simulink model "ASM_Traffic_V2X_Complete_Model_2"  (R2019a)
settings: Solver=ode1  StartTime=SIM.tstart.v  StopTime=Inf  FixedStep=SIM.StepSize.v  RelTol=1e-3
PostLoadFcn:
  | if any(exist('dsrtsu_mdlpostloadfcn', 'file') ~= 0), dsrtsu_mdlpostloadfcn('Execute', bdroot); end
  | try, asm_mdl_postloadfcn(bdroot, 'UpdateModel', 2200); catch, disp(lasterr); end,
undefined symbols (not defined in the file): _SensorPnts_1, _SensorPnts_13, _SensorPnts_17, _SensorPnts_21, _SensorPnts_25, _SensorPnts_29, _SensorPnts_33, _SensorPnts_37, _SensorPnts_41, _SensorPnts_45, _SensorPnts_49, _SensorPnts_5, _SensorPnts_53, _SensorPnts_57, _SensorPnts_9, _to_, CPT, G5A, ITS, MDL, rad, s_to_rpm, SIM
libraries: simulink x169, ASM_VehicleDynamics_lib x126, ASM_Traffic_lib x83, ASM_Utils_lib x49, mdbs x45, ASM_Environment_lib x17, dspindex x12, dsaV2xLibraryAux x10, dsmpblib x6, dsaV2xAsn1Library x4, dsaV2xLibrary x4, ASM_BrakeHydraulics_lib x4
(part 1 of 36)
PreSaveFcn:
  | , if any(exist('dsmpb_private', 'file') ~= 0), dsmpb_private('dsmpb_mdlclblib', 'PreSave', bdroot); end,
CloseFcn:
  | , if any(exist('dsmpb_private', 'file') ~= 0), dsmpb_private('dsmpb_mdlclblib', 'Close', bdroot); end,
settings Model: RTICANMMDATA=struct('GeneralSetupData',struct('modelroot','C:\Users\FHAachenHIL\Desktop\7_DS_Config\5_NoAD_New\1_mdldesk\Simulation\Models','generalsettings',struct('filesettings',struct('destfolder',struct('Name','RTICANMM_FILES','Check',1),'buildfolder',struct('Name','.','Check',1),'AbsDestfolder',struct('Name','C:\Users\FHAachenHIL\Desktop\7_DS_Config\5_NoAD_New\1_mdldesk\Simulation\Models\RTICANMM_FILES'),'AbsBuildfolder',struct('Name','C:\Users\FHAachenHIL\Desktop\7_DS_Config\5_NoAD_New\1_mdldesk\Simulation\Models'))),'options',struct('addpaths',1,'rmpaths',1,'addtrcexclusion',logical(1),'cannavigator',struct('checkmonitoring',0),'show_usrtrc',0,'use_usrtrc',0),'advanced',struct('options',ones(1,100)),'MPSetup',{{}},'RTI',struct('Type','DSRT','Ver','4.1','Date','02-May-2019'),'modelname','ASM_Traffic','block','ASM_Traffic'))  RTILINMMDATA=struct('GeneralSetupData',[])  DSRTSU_INTERNAL_MDBS_VER=10  DSRTSU_INTERNAL_FLEXRAYCONFIG=1  DSRTSU_INTERNAL_RTIFLEXRAYCONFIG=110  DSRTSU_INTERNAL_RTIFPGA=130  DSMPB_DATASERVER_ModelPortLibVersion1=8  DSMPB_DATASERVER_DataServerVersion1=6  DSMPB_DATASERVER_DataServerStreamVersion1=3  DSMPB_ID_DATA={'330216',struct('BlockId','b1f7d386-c077-4b6f-815e-9957a38efec6','SignalIds',{{'5954efed-ef67-4b42-89e3-5084b45090a5','46c6c21c-6ef7-4bce-a685-35314e3aeb42'}}),'330217',struct('BlockId','ed5b6760-6c8b-4597-8985-96cc864119f9','SignalIds',{{'627e4e4b-6795-451d-b132-3b35f692e399','cadb769f-493c-4926-8cfc-80c1d7e415e4'}}),'330693',struct('BlockId','84e11fc7-b113-489b-a36d-07b56c01051e','SignalIds',{{'d6ecdace-abd9-47b0-9636-db978f49e505','b381082d-6ce8-44f4-ad20-a88c694d043c','f1171069-3abf-4521-8686-68da12ae8162','f12997fb-13dd-47fb-a199-884124e88373','33a83d4b-34dd-4bb2-a080-c0d96c0e7444','ed9617ed-63e6-4252-841f-8cd256f9a792','c4d94f54-a4e4-4e6b-a3f5-bdd9f29a9d42','15fc0dc5-818d-41b9-9325-316e0087897d','5fc40cf9-a339-4045-adf5-9eb5a647bd91','2c42badf-67b8-4972-b237-b7d847a79e24','2d6ab885-034a-426b-a4d8-331cba00cc0a','83513bad-946f-4b2a-b06e-a5b54ac67582','7f7e93e0-f84b-4ac0-9920-c275b8003985','b171feba-60b8-420b-b0d7-260006587811','f516aac7-9c5c-4744-8cba-64c96d215c0d','9a91ebe5-1c5e-4056-b557-0e0db1076263','7c50508e-1c47-48c8-9676-4fb8df70f5b9','c6d12e17-68fd-48eb-9242-ce387edb3efa','ff46a663-5f34-440b-b3bc-6b93d7652bc7','70c5629e-94fa-4dad-b003-5f0ee91b30d9','864ca5d3-ee15-40fd-9f67-5bde9bd55b65','8c924b41-9569-4218-92a0-ce33cbab6020'}}),'330694',struct('BlockId','a862b2ce-fdfe-464c-a6f1-ee7d5bbd7d76','SignalIds',{{'f2281447-8dd6-4b87-a3fd-ba757601a6a3','ed6577a0-1bef-4f93-882d-9a91ba3803b9','f5072a04-e2e8-432a-9d22-5e39f1b004c4','f9be402e-ef68-469d-9a5b-51e341e63153','1a6fa1c0-c78d-4bef-9fa9-3949581777f9','434f5ee9-f735-4340-9052-50d203bce394','e2750fce-2507-4a3e-a71c-871616da759c','a78121f1-2d1e-4fc1-9bd3-1e700b95df97','cfd43ada-4b18-4913-87c2-7150350b7745','748ab899-55d6-4599-8033-eefc4cf8692b','9396844c-ddf9-495e-bf4a-e4337b26c01b','5061b213-d7ab-4036-a402-68c9d851f2f7','f74f67c2-0a64-4121-bbfc-28e28bf8e47c','af8173ae-b56e-4181-af22-ab3597f99b45','ab6ffc97-b1da-485b-b261-68785b2ecf74','c89e4028-be19-4be4-8ae4-07a9cfb3f304','45dfa9da-2b41-4994-bfb5-431cbec6d91f','0f4a48ac-0d04-4973-a79b-6dba9191f613','4897f706-738b-48a8-bfa9-4dce5adfb66f','b0c4fe5a-1a55-469a-bfc9-3e5a391b1d28','cee4ed91-4e62-4f16-9db1-8814ccf7c0ec','e77965e1-b7f4-415c-8908-9a91dfd04724','79bd3ed0-ae18-424e-8479-e097ea261fa6','7949adab-96d5-4dfd-97c4-d5cf440e986d','f2ab8de1-88d0-4341-92a1-f4defd2f3f90','bd765ffd-b1df-4d20-b40b-b08ba0baa9bb','147a83a7-172e-4604-bf04-5a0b9f9a69a1','0e989faa-5d6f-437a-9608-bc5915cdfdf7','9a39d9cd-2ac6-4fea-a823-ea5bd99f580f','d9bd35d1-ce0d-4e25-a189-106bd4b9f84a','959e6de5-da96-4cd1-851d-d0057e4456fd','815f072c-0a7f-4fd6-8c30-6c40f700a896','9aee9d69-733b-49cd-a80a-36da2771f58f','c6f90d32-086e-4841-a108-56354959159b','22eea55d-9a77-4830-86d9-89efdace94fd','c76acaa7-4d73-4d33-9929-8168234ee063','008c6442-9318-4b95-b3d4-07b53b0292c2','b9a30481-22be-4824-9a7c-3a367da5f7e5','5e0cc0b3-4c73-42d3-a56f-471d727ce12d','359885a3-4826-4c3f-aa50-e301bb0f4184','d9b051c3-0428-436f-b8e9-eace4c2c4579','64f5c317-cb27-4a4c-a325-cf6357cb844b','7aed38b5-9bc9-415a-b216-13916177e212','02cf0d23-4107-47fd-84c3-b252337a1963','9c33dc05-2142-432c-9611-36045ad6ec16','ecac5224-2058-46c9-8367-a0d51085fe1f','765bb1a7-d023-41a8-903d-a406451af4fc','4f5bc921-bb9b-4516-a2d8-0d46d6edfa0a','0e14b839-d491-4a1e-aee6-f3f5c7d7bb50','18457238-79de-4e3a-b0d5-409821aa4bed','96051f25-1d22-4dec-ba6f-cc499131fb3a','e18ed66a-7425-4928-a383-5204f5397d27','8d75ab57-f5b7-4d53-8d2e-f8c76d8569c5','36687092-25b3-42f9-a75c-3416bb5260bf','4d5e1a10-c54b-4820-9d88-b0136d7cd812','e599ed13-c6b6-48bb-9374-2671a82569d4','e3af4b03-3db2-441e-a0d6-4f276b79ce4b','825e78c5-827a-4970-b8fe-44ed3d477788','2f348dc1-d43d-4671-b1d1-f46cbe87daf1','343e3104-2314-4619-bae1-dd4c090fa7f4','df4bf909-7eb9-4362-a9c5-d81bea227330','98a03783-5fbc-4b9c-9f1c-81a74cb7af6a','78b869f6-02a3-46b3-8c42-971033ba9de4','88004e9a-d91f-47b9-be0c-5672408ac348','189c9c44-5221-417e-8836-60725b723848','af946d2b-57a6-4c2c-b71f-140b6b02e3f2','90df5bec-5be3-41f9-af4b-0493e5795b67','fee887a9-08b2-4953-96dd-4babc6fd5546','380eb70b-fa16-4dfe-9ee9-78d9cb411dc3','8fe8fb63-2564-43be-828c-a9fe295685f8','33c79d6b-d586-49a0-b7f4-4da2ad91c284','ef27260e-aa76-4ab9-ad3c-03633dde9629','16e6a066-1ed3-4b81-aeb3-56afa55c5cd5','b5c7f2f0-3061-4b24-8ee7-62b27506b806','a2f3d904-f536-4b77-b5ff-26007e182bbc','36680f63-c3b8-4f7c-80dd-29cde9b0854b','4673084a-8171-4f71-bcf9-20c0cf4be7ec','9fa3876b-04bc-431e-ad1d-b72f3b83e37a','37709b06-26d1-4f27-8a6e-c8f1f3493499','0a27576c-b094-4959-ae10-24487d3618bf','b94ac14c-7ff3-4bf2-adc1-e7dcf8ef846d','aa040f24-dfe5-430e-9730-a81b7dc3f6ac','90fd4bbc-ec0f-49bd-9db7-b68249f724e1'}}),'331181',struct('BlockId','25fb538d-07fb-4743-a50e-e603533b0f87','SignalIds',{{'5c53568f-464d-4855-ac76-5002436bdbd6','27e61e6d-fb1c-4471-9743-a52ae1b3f7c4'}}),'331182',struct('BlockId','708c40ea-cccc-4db9-ac35-2feb2ef4f622','SignalIds',{{'d81b8d06-2b1c-443c-8694-f188bd9bd534','cf1714a3-1e9a-4a8e-855e-03d4d95ed40a'}})}  ExtModeArmWhenConnect=off  Creator=dSPACE GmbH  LastModifiedBy=FHAachenHIL
settings DataIOCC: SaveFormat=Structure  SignalLoggingSaveFormat=ModelDataLogs  SaveOutput=off  SaveTime=off  ReturnWorkspaceOutputs=off  SignalLoggingName=sigsOut
settings OptimizationCC: BlockReduction=off  BooleanDataType=off  ConditionallyExecuteInputs=off  OptimizeBlockIOStorage=off  BufferReuse=off  GlobalBufferReuse=off  ExpressionFolding=off  ExpressionDepthLimit=2147483647  LocalBlockOutputs=off  InitFltsAndDblsToZero=on  OptimizeDataStoreBuffers=off  BusAssignmentInplaceUpdate=off
settings DebuggingCC: SignalInfNanChecking=warning  SaveWithParameterizedLinksMsg=none  SignalResolutionControl=TryResolveAllWithWarning  InheritedTsInSrcMsg=none  MultiTaskDSMMsg=warning  MultiTaskCondExecSysMsg=none  MultiTaskRateTransMsg=warning  TasksWithSamePriorityMsg=none  CheckMatrixSingularityMsg=warning  FcnCallInpInsideContextMsg=warning  AllowSymbolicDim=off  StateNameClashWarn=warning  StrictBusMsg=ErrorOnBusTreatedAsVector  NonBusSignalsTreatedAsBus=error  SFUnexpectedBacktrackingDiag=warning  SFNoUnconditionalDefaultTransitionDiag=warning  SFExecutionAtInitializationDiag=none  ArithmeticOperatorsInVariantConditions=warning
settings HardwareCC: ProdBitPerPointer=32  ProdBitPerSizeT=32  ProdBitPerPtrDiffT=32  ProdLargestAtomicInteger=Integer  ProdWordSize=32  ProdHWDeviceType=Custom Processor->Custom  TargetIntDivRoundTo=Zero  TargetEndianess=LittleEndian  TargetHWDeviceType=Custom Processor->Custom
settings ModelReferenceCC: PropagateSignalLabelsOutOfModel=off
settings SFSimCC: SimUseLocalCustomCode=off  MATLABDynamicMemAlloc=off
settings RTWCC: SystemTargetFile=dsrt.tlc  GenCodeOnly=on  MakeCommand=make_dsrt  TemplateMakefile=dsrt_default_tmf  Description=dSPACE Run-Time Target (for VEOS and ConfigurationDesk)  RTWVerbose=off  RetainRTWFile=on  RTWUseLocalCustomCode=off
settings CodeAppCC: StateflowObjectComments=on
settings STFCustomTargetCC: ParMdlRefBuildCompliant=on  GRTInterface=off  SystemTargetFile=dsrt.tlc
settings GRTTargetCC: TargetLangStandard=C89/C90 (ANSI)  CompOptLevelCompliant=off  ConcurrentExecutionCompliant=off  CombineOutputUpdateFcns=off  MatFileLogging=off  CPPClassGenCompliant=off  UseToolchainInfoCompliant=off
settings ConfigComp: CovMetricSettings=dw  CovHtmlReporting=on  CovSaveCumulativeToWorkspaceVar=on  CovSaveSingleToWorkspaceVar=on  CovExternalEMLEnable=off  CovSFcnEnable=off

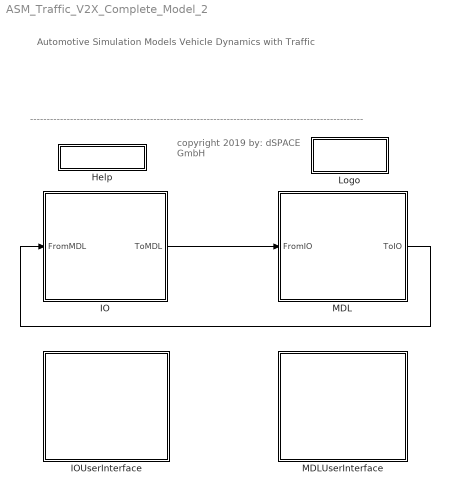
== system ASM_Traffic_V2X_Complete_Model_2 ==
  note: ----------------------------------------------------------------------------------------------------
  note: copyright 2019 by:
      | dSPACE GmbH
  note: Automotive Simulation Models
      | Vehicle Dynamics with Traffic
  Help : Subsystem
      settings: OpenFcn=eval(get_param(gcb,'MaskHelp'))
      mask Help: eval('asm_modelhelp(0,''manual'',''ASMVehicleDynamicsModelDescription.chm'',0)');
      mask Display: fprintf('Help')
  IO : Subsystem
      mask Display: disp('dSPACE\nPeripheral I/O')
  IOUserInterface : Subsystem
      mask Display: disp('User Interface \nfor IO')
  Logo : Subsystem  mask(dSPACE){EmptyParameter=[]}
      mask prompts: EmptyParameter "Mask Parameter 1:"
      settings: OpenFcn=;
      mask Display: image(imread('asm_mdl_dslogo.tif'));
  MDL : Subsystem
      mask Display: disp('Engine + Vehicle\nSimulation Model')
  MDLUserInterface : Subsystem
      mask Display: disp('User Interface \nfor Model')
  wires:
  MDL/1(ToIO) -> IO/1(FromMDL)
  IO/1(ToMDL) -> MDL/1(FromIO)

== system ASM_Traffic_V2X_Complete_Model_2/Help ==
  note: This library can be used for incylinder diesel engine modeling.

== system ASM_Traffic_V2X_Complete_Model_2/IO ==
  FromMDL : Inport
  I/O_Subsystem : Subsystem
      mask Display: image('can2.jpg');
  V2X_Subsystem : Subsystem
      mask Display: image('v2x.jpg');
  ToMDL : Outport
  wires:
  FromMDL/1 -> I/O_Subsystem/1(In1), V2X_Subsystem/1(In1)
  I/O_Subsystem/1(Out1) -> ToMDL/1

== system ASM_Traffic_V2X_Complete_Model_2/IOUserInterface ==
  IO_DISP : Subsystem
      mask Display: disp('Simulation results:\nArbitrary input to\nControlDesk from I/O')
  IO_PAR : Subsystem
      mask Display: disp('Simulation parameters:\nContinuous output from\nControlDesk to I/O')

== system ASM_Traffic_V2X_Complete_Model_2/Logo ==
  note: $Revision: 1.234 $
  note: $Date: 2014/11/26 16:23:07MEZ $
  note: $Workfile: ASM_VehicleDynamics.mdl $

== system ASM_Traffic_V2X_Complete_Model_2/MDL ==
  FromIO : Inport
  Drivetrain : Subsystem
  Engine : Subsystem
  Environment : Subsystem
  MDL_In : Subsystem
  MDL_Out : Subsystem
  SoftECU : Subsystem
  VehicleDynamics : Subsystem
  ToIO : Outport
  wires:
  SoftECU/1(SoftECU_Signals) -> MDL_In/1(from_SoftECU)
  MDL_Out/1(to_IO) -> Environment/1(Vehicle_Signals), SoftECU/1(Vehicle_Signals), ToIO/1
  FromIO/1 -> Environment/2(Input), MDL_In/2(from_IO)
  VehicleDynamics/1(omega_Wheel[FL,FR,RL,RR][rad|s]) -> Drivetrain/3(omega_Wheel[FL,FR,RL,RR][rad|s])
  Drivetrain/2(Trq_Shaft[FL,FR,RL,RR][Nm]) -> VehicleDynamics/1(Trq_Shaft[FL,FR,RL,RR][Nm])
  Engine/1(Trq_Engine[Nm]) -> Drivetrain/1(Trq_Engine[Nm])
  Drivetrain/1(n_Engine[rpm]) -> Engine/2(n_Engine[rpm])
  Environment/1(Environment_Signals) -> VehicleDynamics/2(Environment_Signals), Engine/1(Environment_Signals), SoftECU/2(Environment_Signals), Drivetrain/2(Environment_Signals)

== system ASM_Traffic_V2X_Complete_Model_2/MDLUserInterface ==
  note: --------------------------------- Display Signals and Change Parameters ----------------------------------------------------------------------------------------------------------------------
  note: ----------------------------------------------- MotionDesk 3D-Animation ------------------------------------------------------------
  note: For MotionDesk support replace this block  with the MotionDesk
      | interface from the "ASM_MotionDeskInterface.mdl" which
      | can be found in the "Models" directory.
  note: -------------------- Scope Handling ----------------------
  note: --- Tire Handling ---
  note: --------- Developer/Operator Handling ----------
  note: ----------------------- Project & Experiment Handling -------------------------
  note: ------- Code Generation -------
  note: --- ModelDesk Parameter Group ---
  note: ------- Multi-Instance -------
  ActivateDeveloperVersion : ASM_Utils_lib/Operator/ActivateDeveloperVersion  plotblock_updt=0
  ActivateOperatorVersion : ASM_Utils_lib/Operator/ActivateOperatorVersion  plotblock_updt=0
  Drivetrain : Subsystem
      mask Display: disp('Drivetrain');
  Engine : Subsystem
      mask Display: disp('Engine');
  Environment : Subsystem
      mask Display: disp('Environment');
  GenerateVEOS : ASM_Utils_lib/CodeGeneration/GenerateVEOS
  ModelDeskParaGroupOverview : ASM_Utils_lib/ModelDeskInterface/ModelDeskParaGroupOverview
  ModelDesk_Plotting : Subsystem  Tag=ModelDeskPlottingInterface
      mask Display: disp('ModelDesk Plotting');
  MotionDeskInterface : Subsystem  Tag=MotionDeskInterface
      mask Display: disp('MotionDesk Interface\nSet Configuration Parameters Inside')
  MultiInstanceOverview : ASM_Utils_lib/ModelDeskInterface/MultiInstanceOverview
  OpenExperiment1 : ASM_Utils_lib/OpenExperiment/OpenExperiment  ExpDir=..\Animation\MotionDesk_Traffic\ASMTraffic\ASMTraffic.mdd  dSProduct=MotionDesk
  OpenExperiment2 : ASM_Utils_lib/OpenExperiment/OpenExperiment  ExpDir=..\Parameterization\MOD_Traffic\Experiment_001\Experiment_001.CDE  dSProduct=ModelDesk
  OpenMotionDeskInterfaceModel : Subsystem
      settings: OpenFcn=|
      | InterfaceModel = 'ASM_MotionDeskInterface';
      | 
      | try
      |     open_system(InterfaceModel);                         catch
      |     errordlg(['ERROR opening MotionDesk interface: ',InterfaceModel,'.mdl.']);
      | end
      mask Display: disp('Open\nASM_MotionDeskInterface\nModel')
  ReplaceTireTMEasy : ASM_Utils_lib/BlockReplacement/ReplaceTireTMEasy
  ScopeHandlingGui : ASM_Utils_lib/ReplaceScopes/ScopeHandlingGui
  SoftECU : Subsystem
      mask Display: disp('Soft ECU');
  Toggle_ModelDesk_Plotting : MDLD_Utils_lib/ModelDeskPlotInterface/Toggle_ModelDesk_Plotting  SystemSampleTime=-1
  VehicleDynamics : Subsystem
      mask Display: disp('Vehicle Dynamics');

== system ASM_Traffic_V2X_Complete_Model_2/IO/I//O_Subsystem ==
  note: EGO CAR DATA for CONTROL PC CAN BUS
  note: CAN BUS DATA from CONTROL PC to EGO CAR
  In1 : Inport
  Bus Configuration (1) - In : Subsystem
  Bus Configuration (1) - Out : Subsystem
  Bus Configuration (1)_In : dsmpblib/Data Inport  Priority=10000
      settings: SourceProductName=dSPACE Model Interface Blockset
  Bus Configuration (1)_Out : dsmpblib/Data Outport  Priority=-10000
      settings: SourceProductName=dSPACE Model Interface Blockset
  EgoCar_Command : Subsystem
  EgoCar_Data : Subsystem
  Out1 : Outport
  wires:
  In1/1 -> EgoCar_Data/1(In1), EgoCar_Command/2(In2)
  Bus Configuration (1)_In/1 -> Bus Configuration (1) - Out/1(Out), EgoCar_Command/1(In1)
  EgoCar_Command/1(Out1) -> Out1/1
  Bus Configuration (1) - In/1(In) -> Bus Configuration (1)_Out/1
  EgoCar_Data/1(Out1) -> Bus Configuration (1) - In/1(Input)

== system ASM_Traffic_V2X_Complete_Model_2/IO/V2X_Subsystem ==
  In1 : Inport
  CAM-DENM_Message_Generation : Subsystem
  Car_Data : Subsystem
  Subsystem : Subsystem
  wires:
  Car_Data/1(Output) -> CAM-DENM_Message_Generation/1(Input)
  In1/1 -> Subsystem/1(In1), Car_Data/1(Fellow_Pos_info)

== system ASM_Traffic_V2X_Complete_Model_2/IOUserInterface/IO_DISP ==

== system ASM_Traffic_V2X_Complete_Model_2/IOUserInterface/IO_PAR ==

== system ASM_Traffic_V2X_Complete_Model_2/MDL/Drivetrain ==
  Trq_Engine[Nm] : Inport
  Environment_Signals : Inport  Port=2
  omega_Wheel[FL,FR,RL,RR][rad|s] : Inport  Port=3
  ASMSignalCollector : Subsystem
  Bus Selector1 : BusSelector  OutputSignals=Maneuver.Testbench.n_Engine_Set[rpm],Maneuver.Testbench.SW_Testbench[0Off|1On],Driver.Pos_ClutchPedal[%],Driver.Gear[],Maneuver.MdlControl.Reset_VehicleStates[0|1]
  Bus Selector2 : BusSelector  OutputSignals=Sw_AC[0|1],Ctrl_Lockup_Clutch[%],Gear[]
  Bus Selector3 : BusSelector  OutputSignals=Sw_Starter[0Off|1On]
  Crankshaft : Subsystem  Tag=ASM_CRANKSHAFT
      settings: CopyFcn=asm_blk_copy_gui('start','usecase','crankshaftcopy','drivetrain_variant','flexible')
  DisableReset : Subsystem
      mask Display: disp('DisableReset')
  External Loads : Subsystem
  Final_Drive_Assembly : Subsystem  Tag=ASM_FINAL_DRIVE_ASSEMBLY
      settings: CopyFcn=asm_blk_copy_gui('start','usecase','finaldrivecopy','drivetrain_variant','flexible')
  ModelDesk_MC_ID_Drivetrain : ASM_Utils_lib/ModelDeskInterface/ModelDesk_MC_ID_Drivetrain  Tag=ASM_MAINCOMPONENT  ASMProperties=struct('Name','Drivetrain')
  OpenCrankshaftDemos : Subsystem
      settings: OpenFcn=asm_open_lib('ASM_VehicleDynamics_lib/Drivetrain/Demos_Crankshaft');
      mask Display: disp('Open Demos\nCrankshaft')
  OpenFinalDriveAssemblyDemos : Subsystem
      settings: OpenFcn=asm_open_lib('ASM_VehicleDynamics_lib/Drivetrain/Demos_Final_Drive_Assembly');
      mask Display: disp('Open Demos\nFinal Drive Assembly')
  OpenTransmissionSystemDemos : Subsystem
      settings: OpenFcn=asm_open_lib('ASM_VehicleDynamics_lib/Drivetrain/Demos_Transmission_System');
      mask Display: disp('Open Demos\nTransmission System')
  STARTER : ASM_VehicleDynamics_lib/Drivetrain/Crankshaft_and_Starter/STARTER  Tag=ASM_SUBCOMPONENT  Const_Trq_n0=MDL.Drivetrain.Starter.Const_Trq_n0  Const_n_Trq0=MDL.Drivetrain.Starter.Const_n_Trq0  Const_Inertia_Starter=MDL.Drivetrain.Starter.Const_Inertia_Starter  ASMProperties=struct('Name','STARTER','Version','4.0','Library','ASM_VehicleDynamics_lib')  ASMInstanceName=starter  ASMInstanceID=1
  TEST_BENCH : ASM_VehicleDynamics_lib/Drivetrain/Crankshaft_and_Starter/TEST_BENCH  Tag=ASM_SUBCOMPONENT  Const_P_Gain=MDL.Drivetrain.TestBench.Const_P_Gain  Const_I_Gain=MDL.Drivetrain.TestBench.Const_I_Gain  Const_Trq_Max_TestBench=MDL.Drivetrain.TestBench.Const_Trq_Max_TestBench  Const_Inertia_TestBench=MDL.Drivetrain.TestBench.Const_Inertia_TestBench  StepSize=SIM.StepSize  ASMProperties=struct('Name','TEST_BENCH','Version','2.0','Library','ASM_VehicleDynamics_lib')  ASMInstanceName=test_bench  ASMInstanceID=1
  Transmission : Subsystem  Tag=ASM_TRANSMISSION
      settings: CopyFcn=asm_blk_copy_gui('start','usecase','transmissioncopy','drivetrain_variant','flexible')
  n_Engine[rpm] : Outport
  Trq_Shaft[FL,FR,RL,RR][Nm] : Outport  Port=2
  tag scope: ASMBUS_Drivetrain_Starter=global, ASMBUS_Drivetrain_Test_Bench=global
  wires:
  External Loads/1(Trq_External[Nm]) -> Crankshaft/2(Trq_External[Nm])
  External Loads/2(Intertia_External[kgm2]) -> Crankshaft/3(Inertia_External[kgm2])
  DisableReset/1(Reset[0|1]) -> Crankshaft/4(Reset[0|1]), Transmission/8(Reset[0|1])
  TEST_BENCH/3 -> External Loads/1(Inertia_TestBench[kgm2])
  TEST_BENCH/1 -> [ASMBUS_Drivetrain_Test_Bench]
  Bus Selector3/1 -> STARTER/1  "<Sw_Starter[0Off|1On]>"
  [TAG_FromIO_Engine] -> Bus Selector3/1
  TEST_BENCH/2 -> Crankshaft/1(Trq_TestBench[Nm])
  Transmission/3(Trq_Out_Trm[Nm]) -> Final_Drive_Assembly/2(Trq_Out_Trm[Nm])
  Transmission/2(Inertia_Out_Trm[kgm2]) -> Final_Drive_Assembly/1(Inertia_Trm[kgm2])
  Final_Drive_Assembly/1(omega_In_Diff[rad|s]) -> Transmission/9(omega_In_Diff[rad|s])
  STARTER/1 -> [ASMBUS_Drivetrain_Starter]
  Bus Selector2/1 -> External Loads/4(Sw_AC[0|1])  "<Sw_AC[0|1]>"
  Bus Selector1/2 -> TEST_BENCH/3  "<SW_Testbench[0Off|1On]>"
  Bus Selector1/1 -> TEST_BENCH/2  "<n_Engine_Set[rpm]>"
  STARTER/2 -> External Loads/2(Trq_Starter[Nm])
  STARTER/3 -> External Loads/3(Inertia_Starter[kgm2])
  Transmission/1(Trq_Fric[Nm]) -> Crankshaft/6(Trq_Fric_Clutch[Nm])
  [TAG_Sw_Transmission_Mode] -> Transmission/7(SW_TrmMode[1Manual|2Automatic])
  Bus Selector2/2 -> Transmission/3(Ctrl_Lockup_Clutch[%])  "<Ctrl_Lockup_Clutch[%]>"
  Bus Selector2/3 -> Transmission/4(Gear_AT[])  "<Gear[]>"
  Bus Selector1/3 -> Transmission/5(Pos_ClutchPedal_MT[%])  "<Pos_ClutchPedal[%]>"
  Bus Selector1/4 -> Transmission/6(Gear_MT[])  "<Gear[]>"
  Bus Selector1/5 -> Final_Drive_Assembly/3(Reset[0|1]), DisableReset/1(Reset_VehicleStates[0|1]), TEST_BENCH/4  "<Reset_VehicleStates[0|1]>"
  Crankshaft/2(n_Engine[rad|s]) -> Transmission/2(n_Engine[rad|s])
  omega_Wheel[FL,FR,RL,RR][rad|s]/1 -> Final_Drive_Assembly/4(omega_Wheel[FL,FR,RL,RR][rad|s])
  [TAG_FromIO_Drivetrain] -> Bus Selector2/1
  Trq_Engine[Nm]/1 -> Crankshaft/5(Trq_Engine[Nm]), Transmission/1(Trq_Engine[Nm])
  Crankshaft/1(n_Engine[rpm]) -> TEST_BENCH/1, STARTER/2, n_Engine[rpm]/1
  Final_Drive_Assembly/2(Trq_Shaft[FL,FR,RL,RR][Nm]) -> Trq_Shaft[FL,FR,RL,RR][Nm]/1
  Environment_Signals/1 -> Bus Selector1/1

== system ASM_Traffic_V2X_Complete_Model_2/MDL/Engine ==
  Environment_Signals : Inport
  n_Engine[rpm] : Inport  Port=2
  ASMSignalCollector : Subsystem
  Bus Selector : BusSelector  OutputSignals=Maneuver.MdlControl.Reset_VehicleStates[0|1]
  Bus Selector1 : BusSelector  OutputSignals=Pos_AccPedal_Influenced[%],Pos_AccPedal_Driver_Des[%],Engine_Dynamic_Fast[0|1]
  Bus Selector2 : BusSelector  OutputSignals=Trq_Ind_Engine[Nm]
  ENGINE : ASM_VehicleDynamics_lib/EngineBasic/ENGINE  Tag=ASM_SUBCOMPONENT  Map_Torque=MDL.EngineBasic.Engine.Map_Trq_MeanEff_Engine  Const_TimeConst_Increase=MDL.EngineBasic.Engine.Const_TimeConst_Increase  Const_TimeConst_Decrease=MDL.EngineBasic.Engine.Const_TimeConst_Decrease  Const_TimeConst_Fast=MDL.EngineBasic.Engine.Const_TimeConst_Fast  StepSize=SIM.StepSize  ASMProperties=struct('Name','ENGINE','Version','8.0','Library','ASM_VehicleDynamics_lib')  ASMInstanceName=engine  ASMInstanceID=1
  FUEL_CONSUMPTION : ASM_VehicleDynamics_lib/EngineBasic/FUEL_CONSUMPTION  Tag=ASM_SUBCOMPONENT  Const_rho_Fuel=MDL.EngineBasic.FuelConsumption.Const_rho_Fuel  Map_Specif_FuelConsumption=MDL.EngineBasic.FuelConsumption.Map_Specif_FuelConsumption  Const_Specif_Emission_CO2=MDL.EngineBasic.FuelConsumption.Const_Specif_Emission_CO2  Const_V_Displ=MDL.EngineBasic.FuelConsumption.Const_V_Displ  Const_i=MDL.EngineBasic.FuelConsumption.Const_i  Const_Q_LHV=MDL.EngineBasic.FuelConsumption.Const_Q_LHV  Const_mdot_Fuel_Idle=MDL.EngineBasic.FuelConsumption.Const_mdot_Fuel_Idle  Const_Trq_Fric_Engine_Idle=MDL.EngineBasic.FuelConsumption.Const_Trq_Fric_Engine_Idle  StepSize=SIM.StepSize  ASMProperties=struct('Name','FUEL_CONSUMPTION','Version','2.0','Library','ASM_VehicleDynamics_lib')  ASMInstanceName=fuel_consumption  ASMInstanceID=1
  ModelDesk_MC_ID_EngineBasic : ASM_Utils_lib/ModelDeskInterface/ModelDesk_MC_ID_EngineBasic  Tag=ASM_MAINCOMPONENT  ASMProperties=struct('Name','EngineBasic')
  Terminator : Terminator
  Terminator1 : Terminator
  Terminator2 : Terminator
  Trq_Engine[Nm] : Outport
  tag scope: ASMBUS_EngineBasic_EngineBasic=global, ASMBUS_EngineBasic_FuelConsumption=global
  wires:
  FUEL_CONSUMPTION/1 -> [ASMBUS_EngineBasic_FuelConsumption]
  Bus Selector2/1 -> FUEL_CONSUMPTION/3  "<Trq_Ind_Engine[Nm]>"
  [ASMBUS_EngineBasic_EngineBasic] -> Bus Selector2/1
  FUEL_CONSUMPTION/2 -> Terminator/1
  FUEL_CONSUMPTION/3 -> Terminator1/1
  FUEL_CONSUMPTION/4 -> Terminator2/1
  Environment_Signals/1 -> Bus Selector/1
  ENGINE/1 -> [ASMBUS_EngineBasic_EngineBasic]
  [TAG_FromIO_Engine] -> Bus Selector1/1
  ENGINE/2 -> Trq_Engine[Nm]/1, FUEL_CONSUMPTION/1
  Bus Selector/1 -> ENGINE/5, FUEL_CONSUMPTION/4  "<Reset_VehicleStates[0|1]>"
  n_Engine[rpm]/1 -> ENGINE/1, FUEL_CONSUMPTION/2
  Bus Selector1/1 -> ENGINE/2  "<Pos_AccPedal_Influenced[%]>"
  Bus Selector1/2 -> ENGINE/3  "<Pos_AccPedal_Driver_Des[%]>"
  Bus Selector1/3 -> ENGINE/4  "<Engine_Dynamic_Fast[0|1]>"

== system ASM_Traffic_V2X_Complete_Model_2/MDL/Environment ==
  Vehicle_Signals : Inport
  Input : Inport  Port=2
  ASMSignalCollector : Subsystem
  Bus Creator : BusCreator  Inputs=4
  Driver : Subsystem
  EnvironmentInterface_In : Subsystem
  Maneuver : Subsystem
  ModelDesk_MC_ID_Environment : ASM_Utils_lib/ModelDeskInterface/ModelDesk_MC_ID_Environment  Tag=ASM_MAINCOMPONENT  ASMProperties=struct('Name','Environment')
  Road : Subsystem
  Traffic : Subsystem
  Environment_Signals : Outport
  wires:
  EnvironmentInterface_In/3(SoftECU_Signals) -> Maneuver/5(SoftECU_Signals), Driver/5(SoftECU_Engine_Signals)
  Bus Creator/1 -> Environment_Signals/1
  Driver/2(s_Preview[m]) -> Road/1(s_Preview[m])
  Maneuver/1(Maneuver_Signals) -> Traffic/2(Maneuver_Signals), Road/2(Maneuver_Signals), Driver/2(Maneuver_Signals), Bus Creator/1
  Road/1(Road_Signals) -> Bus Creator/3, Maneuver/1(Road_Signals), Driver/1(Road_Signals), Traffic/1(Road_Signals)
  Driver/1(Driver_Signals) -> Maneuver/3(Driver_Signals), Bus Creator/2
  Vehicle_Signals/1 -> EnvironmentInterface_In/1(Vehicle_Signals)
  EnvironmentInterface_In/1(VehicleDynamics_Signals) -> Driver/3(VehicleDynamics_Signals), Traffic/3(VehicleDynamics_Signals), Road/3(VehicleDynamics_Signals), Maneuver/2(VehicleDynamics_Signals)
  EnvironmentInterface_In/2(Drivetrain_Signals) -> Driver/4(Drivetrain_Signals)
  Traffic/2(Traffic_Signals) -> Maneuver/4(Traffic_Signals), Bus Creator/4
  Traffic/1(Traffic_Signals_toRoad) -> Road/4(Traffic_Signals)
  Input/1 -> Driver/6(Input)

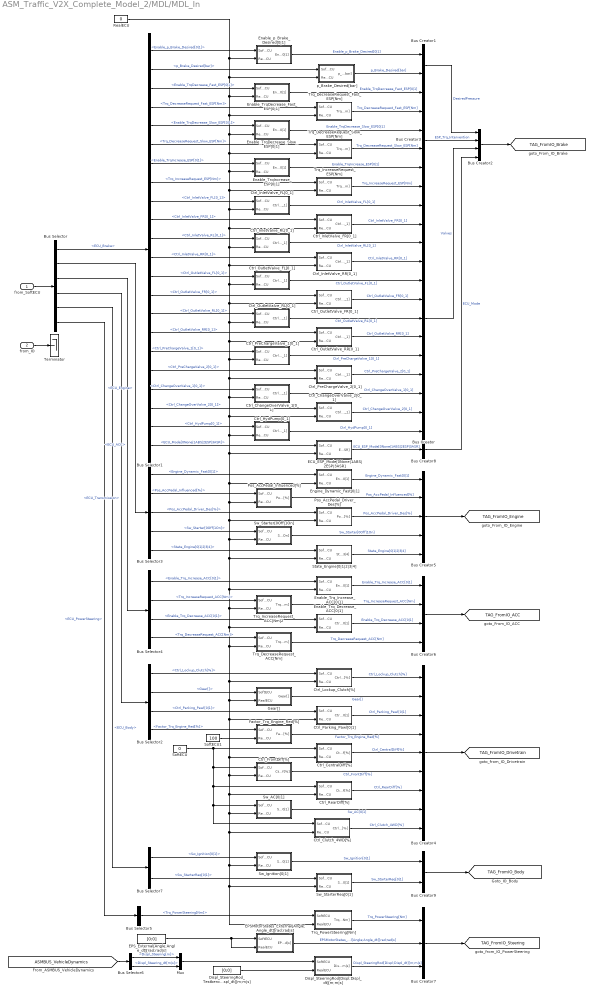
== system ASM_Traffic_V2X_Complete_Model_2/MDL/MDL_In ==
  from_SoftECU : Inport
  from_IO : Inport  Port=2
  Bus Creator : BusCreator  Inputs=13
  Bus Creator1 : BusCreator  Inputs=2
  Bus Creator2 : BusCreator  Inputs=4
  Bus Creator3 : BusCreator  Inputs=6
  Bus Creator4 : BusCreator  Inputs=9
  Bus Creator5 : BusCreator  Inputs=5
  Bus Creator6 : BusCreator  Inputs=4
  Bus Creator7 : BusCreator  Inputs=3
  Bus Creator8 : BusCreator  Inputs=1
  Bus Creator9 : BusCreator  Inputs=2
  Bus Selector : BusSelector  OutputSignals=ECU_Brake,ECU_Engine,ECU_ACC,ECU_Transmission,ECU_Body,ECU_PowerSteering
  Bus Selector1 : BusSelector  OutputSignals=Enable_p_Brake_Desired[0|1],p_Brake_Desired[bar],Trq_Intervention.Enable_TrqDecrease_Fast_ESP[0|1],Trq_Intervention.Trq_DecreaseRequest_Fast_ESP[Nm],Trq_Intervention.Enable_TrqDecrease_Slow_ESP[0|1],Trq_Intervention.Trq_DecreaseRequest_Slow_ESP[Nm],Trq_Intervention.Enable_TrqIncrease_ESP[0|1],Trq_Intervention.Trq_IncreaseRequest_ESP[Nm],Valves.Ctrl_InletValve_FL[0_1],Valves.Ctrl_InletValve_FR[0_1],Valves.Ctrl_InletValve_RL[0_1],Valves.Ctrl_InletValve_RR[0_1],Valves.Ctrl_OutletValve_FL[0_1],Valves.Ctrl_OutletValve_FR[0_1],Valves.Ctrl_OutletValve_RL[0_1],Valves.Ctrl_OutletValve_RR[0_1],Valves.Ctrl_PreChargeValve_1[0_1],Valves.Ctrl_PreChargeValve_2[0_1],Valves.Ctrl_ChangeOverValve_1[0_1],Valves.Ctrl_ChangeOverValve_2[0_1],Valves.Ctrl_HydPump[0_1],ECU_Mode[0None|1ABS|2ESP|3ASR]
  Bus Selector2 : BusSelector  OutputSignals=Ctrl_Lockup_Clutch[%],Gear[],Ctrl_Parking_Pawl[0|1],Factor_Trq_Engine_Red[%]
  Bus Selector3 : BusSelector  OutputSignals=Engine_Dynamic_Fast[0|1],Pos_AccPedal_Influenced[%],Pos_AccPedal_Driver_Des[%],Sw_Starter[0Off|1On],State_Engine[0|1|2|3|4]
  Bus Selector4 : BusSelector  OutputSignals=Enable_Trq_Increase_ACC[0|1],Trq_IncreaseRequest_ACC[Nm],Enable_Trq_Decrease_ACC[0|1],Trq_DecreaseRequest_ACC[Nm]
  Bus Selector5 : BusSelector  OutputSignals=Trq_PowerSteering[Nm]
  Bus Selector6 : BusSelector  OutputSignals=Steering.Displ_Steering[m],Steering.Displ_Steering_dt[m|s]
  Bus Selector7 : BusSelector  OutputSignals=Sw_Ignition[0|1],Sw_StarterReq[0|1]
  Ctrl_CentralDiff[%] : Subsystem
  Ctrl_ChangeOverValve_1[0_1] : Subsystem
  Ctrl_ChangeOverValve_2[0_1] : Subsystem
  Ctrl_Clutch_4WD[%] : Subsystem
  Ctrl_FrontDiff[%] : Subsystem
  Ctrl_HydPump[0_1] : Subsystem
  Ctrl_InletValve_FL[0_1] : Subsystem
  Ctrl_InletValve_FR[0_1] : Subsystem
  Ctrl_InletValve_RL[0_1] : Subsystem
  Ctrl_InletValve_RR[0_1] : Subsystem
  Ctrl_Lockup_Clutch[%] : Subsystem
  Ctrl_OutletValve_FL[0_1] : Subsystem
  Ctrl_OutletValve_FR[0_1] : Subsystem
  Ctrl_OutletValve_RL[0_1] : Subsystem
  Ctrl_OutletValve_RR[0_1] : Subsystem
  Ctrl_Parking_Pawl[0|1] : Subsystem
  Ctrl_PreChargeValve_1[0_1] : Subsystem
  Ctrl_PreChargeValve_2[0_1] : Subsystem
  Ctrl_RearDiff[%] : Subsystem
  Displ_SteeringRod[Displ;Displ_dt][m;m|s] : Subsystem
  Displ_SteeringRod_Testbench[Displ;Displ_dt][m;m|s] : Constant  Value=[0;0]
  ECU_ESP_Mode[0None|1ABS|2ESP|3ASR] : Subsystem
  EPSMotorStates_External[Angle;Angle_dt][rad;rad|s] : Subsystem
  EPS_External[Angle;Angle_dt][rad;rad|s] : Constant  Value=[0;0]
  Enable_TrqDecrease_Fast_ESP[0|1] : Subsystem
  Enable_TrqDecrease_Slow_ESP[0|1] : Subsystem
  Enable_TrqIncrease_ESP[0|1] : Subsystem
  Enable_Trq_Decrease_ACC[0|1] : Subsystem
  Enable_Trq_Increase_ACC[0|1] : Subsystem
  Enable_p_Brake_Desired[0|1] : Subsystem
  Engine_Dynamic_Fast[0|1] : Subsystem
  Factor_Trq_Engine_Red[%] : Subsystem
  Gear[] : Subsystem
  Mux : Mux  Inputs=2
  Pos_AccPedal_Driver_Des[%] : Subsystem
  Pos_AccPedal_Influenced[%] : Subsystem
  RealECU : Constant  Value=0
  SoftECU : Constant  Value=0
  SoftECU1 : Constant  Value=100
  State_Engine[0|1|2|3|4] : Subsystem
  Sw_AC[0|1] : Subsystem
  Sw_Ignition[0|1] : Subsystem
  Sw_StarterReq[0|1] : Subsystem
  Sw_Starter[0Off|1On] : Subsystem
  Terminator : Terminator
  Trq_DecreaseRequest_ACC[Nm] : Subsystem
  Trq_DecreaseRequest_Fast_ESP[Nm] : Subsystem
  Trq_DecreaseRequest_Slow_ESP[Nm] : Subsystem
  Trq_IncreaseRequest_ACC[Nm]2 : Subsystem
  Trq_IncreaseRequest_ESP[Nm] : Subsystem
  Trq_PowerSteering[Nm] : Subsystem
  p_Brake_Desired[bar] : Subsystem
  tag scope: TAG_FromIO_ACC=global, TAG_FromIO_Body=global, TAG_FromIO_Brake=global, TAG_FromIO_Drivetrain=global, TAG_FromIO_Engine=global, TAG_FromIO_Steering=global
  wires:
  Bus Selector/5 -> Bus Selector7/1  "<ECU_Body>"
  Bus Selector7/1 -> Sw_Ignition[0|1]/1(SoftECU)  "<Sw_Ignition[0|1]>"
  Bus Selector7/2 -> Sw_StarterReq[0|1]/1(SoftECU)  "<Sw_StarterReq[0|1]>"
  Bus Creator9/1 -> [TAG_FromIO_Body]
  Sw_Ignition[0|1]/1(Sw_Ignition[0|1]) -> Bus Creator9/1  "Sw_Ignition[0|1]"
  Sw_StarterReq[0|1]/1(Sw_StarterReq[0|1]) -> Bus Creator9/2  "Sw_StarterReq[0|1]"
  RealECU/1 -> Ctrl_OutletValve_RR[0_1]/2(RealECU), Ctrl_PreChargeValve_2[0_1]/2(RealECU), ECU_ESP_Mode[0None|1ABS|2ESP|3ASR]/2(RealECU), Engine_Dynamic_Fast[0|1]/2(RealECU), Pos_AccPedal_Influenced[%]/2(RealECU), Pos_AccPedal_Driver_Des[%]/2(RealECU), Sw_Starter[0Off|1On]/2(RealECU), State_Engine[0|1|2|3|4]/2(RealECU), Enable_Trq_Increase_ACC[0|1]/2(RealECU), Trq_IncreaseRequest_ACC[Nm]2/2(RealECU), Enable_Trq_Decrease_ACC[0|1]/2(RealECU), Trq_DecreaseRequest_ACC[Nm]/2(RealECU), Ctrl_Lockup_Clutch[%]/2(RealECU), Gear[]/2(RealECU), Ctrl_Parking_Pawl[0|1]/2(RealECU), Ctrl_CentralDiff[%]/2(RealECU), Ctrl_FrontDiff[%]/2(RealECU), Ctrl_RearDiff[%]/2(RealECU), Sw_AC[0|1]/2(RealECU), Ctrl_Clutch_4WD[%]/2(RealECU), Trq_PowerSteering[Nm]/2(RealECU), Sw_StarterReq[0|1]/2(RealECU), Sw_Ignition[0|1]/2(RealECU), Ctrl_HydPump[0_1]/2(RealECU), Ctrl_ChangeOverValve_2[0_1]/2(RealECU), Ctrl_ChangeOverValve_1[0_1]/2(RealECU), Ctrl_PreChargeValve_1[0_1]/2(RealECU), Ctrl_OutletValve_RL[0_1]/2(RealECU), Ctrl_OutletValve_FR[0_1]/2(RealECU), Ctrl_OutletValve_FL[0_1]/2(RealECU), Ctrl_InletValve_RR[0_1]/2(RealECU), Ctrl_InletValve_RL[0_1]/2(RealECU), Ctrl_InletValve_FR[0_1]/2(RealECU), Ctrl_InletValve_FL[0_1]/2(RealECU), Trq_IncreaseRequest_ESP[Nm]/2(RealECU), Enable_TrqIncrease_ESP[0|1]/2(RealECU), Trq_DecreaseRequest_Slow_ESP[Nm]/2(RealECU), Enable_TrqDecrease_Slow_ESP[0|1]/2(RealECU), Trq_DecreaseRequest_Fast_ESP[Nm]/2(RealECU), Enable_TrqDecrease_Fast_ESP[0|1]/2(RealECU), p_Brake_Desired[bar]/2(RealECU), Enable_p_Brake_Desired[0|1]/2(RealECU)
  SoftECU1/1 -> Factor_Trq_Engine_Red[%]/2(RealECU)
  Bus Selector2/4 -> Factor_Trq_Engine_Red[%]/1(SoftECU)  "<Factor_Trq_Engine_Red[%]>"
  Factor_Trq_Engine_Red[%]/1(Factor_Trq_Engine_Red[%]) -> Bus Creator4/4  "Factor_Trq_Engine_Red[%]"
  Bus Selector3/5 -> State_Engine[0|1|2|3|4]/1(SoftECU)  "<State_Engine[0|1|2|3|4]>"
  State_Engine[0|1|2|3|4]/1(State_Engine[0|1|2|3|4]) -> Bus Creator5/5  "State_Engine[0|1|2|3|4]"
  Mux/1 -> Displ_SteeringRod[Displ;Displ_dt][m;m|s]/1(SoftECU)
  Bus Selector6/2 -> Mux/2  "<Displ_Steering_dt[m|s]>"
  Bus Selector6/1 -> Mux/1  "<Displ_Steering[m]>"
  [ASMBUS_VehicleDynamics] -> Bus Selector6/1
  Displ_SteeringRod_Testbench[Displ;Displ_dt][m;m|s]/1 -> Displ_SteeringRod[Displ;Displ_dt][m;m|s]/2(RealECU)
  EPS_External[Angle;Angle_dt][rad;rad|s]/1 -> EPSMotorStates_External[Angle;Angle_dt][rad;rad|s]/2(RealECU), EPSMotorStates_External[Angle;Angle_dt][rad;rad|s]/1(SoftECU)
  Displ_SteeringRod[Displ;Displ_dt][m;m|s]/1(Displ_SteeringRod[Displ;Displ_dt][m;m|s]) -> Bus Creator7/3  "Displ_SteeringRod[Displ;Displ_dt][m;m|s]"
  EPSMotorStates_External[Angle;Angle_dt][rad;rad|s]/1(EPSMotorStates_External[Angle;Angle_dt][rad;rad|s]) -> Bus Creator7/2  "EPSMotorStates_External[Angle;Angle_dt][rad;rad|s]"
  Bus Selector1/22 -> ECU_ESP_Mode[0None|1ABS|2ESP|3ASR]/1(SoftECU)  "<ECU_Mode[0None|1ABS|2ESP|3ASR]>"
  Bus Creator8/1 -> Bus Creator2/4  "ECU_Mode"
  ECU_ESP_Mode[0None|1ABS|2ESP|3ASR]/1(ECU_ESP_Mode[0None|1ABS|2ESP|3ASR]) -> Bus Creator8/1  "ECU_ESP_Mode[0None|1ABS|2ESP|3ASR]"
  Bus Selector3/4 -> Sw_Starter[0Off|1On]/1(SoftECU)  "<Sw_Starter[0Off|1On]>"
  Sw_Starter[0Off|1On]/1(Sw_Starter[0Off|1On]) -> Bus Creator5/4  "Sw_Starter[0Off|1On]"
  Bus Creator7/1 -> [TAG_FromIO_Steering]
  Bus Selector5/1 -> Trq_PowerSteering[Nm]/1(SoftECU)  "<Trq_PowerSteering[Nm]>"
  Trq_PowerSteering[Nm]/1(Trq_PowerSteering[Nm]) -> Bus Creator7/1  "Trq_PowerSteering[Nm]"
  Bus Selector/6 -> Bus Selector5/1  "<ECU_PowerSteering>"
  Ctrl_Clutch_4WD[%]/1(Ctrl_Clutch_4WD[%]) -> Bus Creator4/9  "Ctrl_Clutch_4WD[%]"
  Pos_AccPedal_Driver_Des[%]/1(Pos_AccPedal_Driver_Des[%]) -> Bus Creator5/3  "Pos_AccPedal_Driver_Des[%]"
  Pos_AccPedal_Influenced[%]/1(Pos_AccPedal_Influenced[%]) -> Bus Creator5/2  "Pos_AccPedal_Influenced[%]"
  Engine_Dynamic_Fast[0|1]/1(Engine_Dynamic_Fast[0|1]) -> Bus Creator5/1  "Engine_Dynamic_Fast[0|1]"
  Bus Selector3/3 -> Pos_AccPedal_Driver_Des[%]/1(SoftECU)  "<Pos_AccPedal_Driver_Des[%]>"
  Bus Selector3/2 -> Pos_AccPedal_Influenced[%]/1(SoftECU)  "<Pos_AccPedal_Influenced[%]>"
  Bus Selector3/1 -> Engine_Dynamic_Fast[0|1]/1(SoftECU)  "<Engine_Dynamic_Fast[0|1]>"
  Ctrl_InletValve_FL[0_1]/1(Ctrl_InletValve_FL[0_1]) -> Bus Creator/1  "Ctrl_InletValve_FL[0_1]"
  Ctrl_InletValve_FR[0_1]/1(Ctrl_InletValve_FR[0_1]) -> Bus Creator/2  "Ctrl_InletValve_FR[0_1]"
  Ctrl_InletValve_RL[0_1]/1(Ctrl_InletValve_RL[0_1]) -> Bus Creator/3  "Ctrl_InletValve_RL[0_1]"
  Ctrl_InletValve_RR[0_1]/1(Ctrl_InletValve_RR[0_1]) -> Bus Creator/4  "Ctrl_InletValve_RR[0_1]"
  Ctrl_OutletValve_FL[0_1]/1(Ctrl_OutletValve_FL[0_1]) -> Bus Creator/5  "Ctrl_OutletValve_FL[0_1]"
  Ctrl_OutletValve_FR[0_1]/1(Ctrl_OutletValve_FR[0_1]) -> Bus Creator/6  "Ctrl_OutletValve_FR[0_1]"
  Ctrl_OutletValve_RL[0_1]/1(Ctrl_OutletValve_RL[0_1]) -> Bus Creator/7  "Ctrl_OutletValve_RL[0_1]"
  Ctrl_OutletValve_RR[0_1]/1(Ctrl_OutletValve_RR[0_1]) -> Bus Creator/8  "Ctrl_OutletValve_RR[0_1]"
  Ctrl_PreChargeValve_1[0_1]/1(Ctrl_PreChargeValve_1[0_1]) -> Bus Creator/9  "Ctrl_PreChargeValve_1[0_1]"
  Ctrl_PreChargeValve_2[0_1]/1(Ctrl_PreChargeValve_2[0_1]) -> Bus Creator/10  "Ctrl_PreChargeValve_2[0_1]"
  Ctrl_ChangeOverValve_1[0_1]/1(Ctrl_ChangeOverValve_1[0_1]) -> Bus Creator/11  "Ctrl_ChangeOverValve_1[0_1]"
  Ctrl_ChangeOverValve_2[0_1]/1(Ctrl_ChangeOverValve_2[0_1]) -> Bus Creator/12  "Ctrl_ChangeOverValve_2[0_1]"
  Bus Creator/1 -> Bus Creator2/3  "Valves"
  Ctrl_HydPump[0_1]/1(Ctrl_HydPump[0_1]) -> Bus Creator/13  "Ctrl_HydPump[0_1]"
  Enable_TrqDecrease_Fast_ESP[0|1]/1(Enable_TrqDecrease_Fast[0|1]) -> Bus Creator3/1  "Enable_TrqDecrease_Fast_ESP[0|1]"
  Trq_DecreaseRequest_Slow_ESP[Nm]/1(Trq_DecreaseRequest_Slow[Nm]) -> Bus Creator3/4  "Trq_DecreaseRequest_Slow_ESP[Nm]"
  Enable_TrqIncrease_ESP[0|1]/1(Enable_TrqIncrease[0|1]) -> Bus Creator3/5  "Enable_TrqIncrease_ESP[0|1]"
  Trq_IncreaseRequest_ESP[Nm]/1(Trq_IncreaseRequest[Nm]) -> Bus Creator3/6  "Trq_IncreaseRequest_ESP[Nm]"
  Trq_DecreaseRequest_Fast_ESP[Nm]/1(Trq_DecreaseRequest_Fast[Nm]) -> Bus Creator3/2  "Trq_DecreaseRequest_Fast_ESP[Nm]"
  Bus Creator3/1 -> Bus Creator2/2  "ESP_Trq_Intervention"
  Bus Creator2/1 -> [TAG_FromIO_Brake]
  Enable_TrqDecrease_Slow_ESP[0|1]/1(Enable_TrqDecrease_Slow[0|1]) -> Bus Creator3/3  "Enable_TrqDecrease_Slow_ESP[0|1]"
  from_IO/1 -> Terminator/1
  Ctrl_Lockup_Clutch[%]/1(Ctrl_Lockup_Clutch[%]) -> Bus Creator4/1  "Ctrl_Lockup_Clutch[%]"
  Bus Selector2/1 -> Ctrl_Lockup_Clutch[%]/1(SoftECU)  "<Ctrl_Lockup_Clutch[%]>"
  Bus Selector2/2 -> Gear[]/1(SoftECU)  "<Gear[]>"
  Bus Selector2/3 -> Ctrl_Parking_Pawl[0|1]/1(SoftECU)  "<Ctrl_Parking_Pawl[0|1]>"
  Gear[]/1(Gear[]) -> Bus Creator4/2  "Gear[]"
  Ctrl_Parking_Pawl[0|1]/1(Ctrl_Parking_Pawl[0|1]) -> Bus Creator4/3  "Ctrl_Parking_Pawl[0|1]"
  Ctrl_CentralDiff[%]/1(Ctrl_CentralDiff[%]) -> Bus Creator4/5  "Ctrl_CentralDiff[%]"
  Ctrl_FrontDiff[%]/1(Ctrl_FrontDiff[%]) -> Bus Creator4/6  "Ctrl_FrontDiff[%]"
  Ctrl_RearDiff[%]/1(Ctrl_RearDiff[%]) -> Bus Creator4/7  "Ctrl_RearDiff[%]"
  Sw_AC[0|1]/1(Sw_AC[0|1]) -> Bus Creator4/8  "Sw_AC[0|1]"
  from_SoftECU/1 -> Bus Selector/1
  Bus Selector/4 -> Bus Selector2/1  "<ECU_Transmission>"
  Bus Selector/1 -> Bus Selector1/1  "<ECU_Brake>"
  Bus Selector1/1 -> Enable_p_Brake_Desired[0|1]/1(SoftECU)  "<Enable_p_Brake_Desired[0|1]>"
  Bus Selector1/2 -> p_Brake_Desired[bar]/1(SoftECU)  "<p_Brake_Desired[bar]>"
  Bus Selector1/3 -> Enable_TrqDecrease_Fast_ESP[0|1]/1(SoftECU)  "<Enable_TrqDecrease_Fast_ESP[0|1]>"
  Bus Selector1/4 -> Trq_DecreaseRequest_Fast_ESP[Nm]/1(SoftECU)  "<Trq_DecreaseRequest_Fast_ESP[Nm]>"
  Enable_p_Brake_Desired[0|1]/1(Enable_p_Brake_Desired[0|1]) -> Bus Creator1/1  "Enable_p_Brake_Desired[0|1]"
  p_Brake_Desired[bar]/1(p_Brake_Desired[bar]) -> Bus Creator1/2  "p_Brake_Desired[bar]"
  Bus Creator1/1 -> Bus Creator2/1  "DesiredPressure"
  Bus Selector1/5 -> Enable_TrqDecrease_Slow_ESP[0|1]/1(SoftECU)  "<Enable_TrqDecrease_Slow_ESP[0|1]>"
  Bus Selector1/6 -> Trq_DecreaseRequest_Slow_ESP[Nm]/1(SoftECU)  "<Trq_DecreaseRequest_Slow_ESP[Nm]>"
  Bus Selector1/7 -> Enable_TrqIncrease_ESP[0|1]/1(SoftECU)  "<Enable_TrqIncrease_ESP[0|1]>"
  Bus Selector1/8 -> Trq_IncreaseRequest_ESP[Nm]/1(SoftECU)  "<Trq_IncreaseRequest_ESP[Nm]>"
  Bus Selector1/9 -> Ctrl_InletValve_FL[0_1]/1(SoftECU)  "<Ctrl_InletValve_FL[0_1]>"
  Bus Selector1/10 -> Ctrl_InletValve_FR[0_1]/1(SoftECU)  "<Ctrl_InletValve_FR[0_1]>"
  Bus Selector1/11 -> Ctrl_InletValve_RL[0_1]/1(SoftECU)  "<Ctrl_InletValve_RL[0_1]>"
  Bus Selector1/12 -> Ctrl_InletValve_RR[0_1]/1(SoftECU)  "<Ctrl_InletValve_RR[0_1]>"
  Bus Selector1/13 -> Ctrl_OutletValve_FL[0_1]/1(SoftECU)  "<Ctrl_OutletValve_FL[0_1]>"
  Bus Selector1/14 -> Ctrl_OutletValve_FR[0_1]/1(SoftECU)  "<Ctrl_OutletValve_FR[0_1]>"
  Bus Selector1/15 -> Ctrl_OutletValve_RL[0_1]/1(SoftECU)  "<Ctrl_OutletValve_RL[0_1]>"
  Bus Selector1/16 -> Ctrl_OutletValve_RR[0_1]/1(SoftECU)  "<Ctrl_OutletValve_RR[0_1]>"
  Bus Selector1/17 -> Ctrl_PreChargeValve_1[0_1]/1(SoftECU)  "<Ctrl_PreChargeValve_1[0_1]>"
  Bus Selector1/18 -> Ctrl_PreChargeValve_2[0_1]/1(SoftECU)  "<Ctrl_PreChargeValve_2[0_1]>"
  Bus Selector1/19 -> Ctrl_ChangeOverValve_1[0_1]/1(SoftECU)  "<Ctrl_ChangeOverValve_1[0_1]>"
  Bus Selector1/20 -> Ctrl_ChangeOverValve_2[0_1]/1(SoftECU)  "<Ctrl_ChangeOverValve_2[0_1]>"
  Bus Selector1/21 -> Ctrl_HydPump[0_1]/1(SoftECU)  "<Ctrl_HydPump[0_1]>"
  Bus Selector/2 -> Bus Selector3/1  "<ECU_Engine>"
  Bus Creator5/1 -> [TAG_FromIO_Engine]
  Bus Selector/3 -> Bus Selector4/1  "<ECU_ACC>"
  Bus Selector4/1 -> Enable_Trq_Increase_ACC[0|1]/1(SoftECU)  "<Enable_Trq_Increase_ACC[0|1]>"
  Bus Selector4/2 -> Trq_IncreaseRequest_ACC[Nm]2/1(SoftECU)  "<Trq_IncreaseRequest_ACC[Nm]>"
  Bus Selector4/3 -> Enable_Trq_Decrease_ACC[0|1]/1(SoftECU)  "<Enable_Trq_Decrease_ACC[0|1]>"
  Bus Selector4/4 -> Trq_DecreaseRequest_ACC[Nm]/1(SoftECU)  "<Trq_DecreaseRequest_ACC[Nm]>"
  Enable_Trq_Increase_ACC[0|1]/1(Enable_Trq_Increase_ACC[0|1]) -> Bus Creator6/1  "Enable_Trq_Increase_ACC[0|1]"
  Trq_IncreaseRequest_ACC[Nm]2/1(Trq_IncreaseRequest_ACC[Nm]) -> Bus Creator6/2  "Trq_IncreaseRequest_ACC[Nm]"
  Enable_Trq_Decrease_ACC[0|1]/1(Ctrl_ChangeOverValve_2[0|1]) -> Bus Creator6/3  "Enable_Trq_Decrease_ACC[0|1]"
  Trq_DecreaseRequest_ACC[Nm]/1(Trq_DecreaseRequest_ACC[Nm]) -> Bus Creator6/4  "Trq_DecreaseRequest_ACC[Nm]"
  Bus Creator6/1 -> [TAG_FromIO_ACC]
  Bus Creator4/1 -> [TAG_FromIO_Drivetrain]
  SoftECU/1 -> Ctrl_CentralDiff[%]/1(SoftECU), Ctrl_FrontDiff[%]/1(SoftECU), Sw_AC[0|1]/1(SoftECU), Ctrl_Clutch_4WD[%]/1(SoftECU), Ctrl_RearDiff[%]/1(SoftECU)

== system ASM_Traffic_V2X_Complete_Model_2/MDL/MDL_Out ==
  Bus Creator : BusCreator  Inputs=5
  to_IO : Outport
  tag scope: ASMBUS_Complete=global
  wires:
  [ASMBUS_SoftECU] -> Bus Creator/1
  Bus Creator/1 -> [ASMBUS_Complete], to_IO/1
  [ASMBUS_Environment] -> Bus Creator/5
  [ASMBUS_Drivetrain] -> Bus Creator/4
  [ASMBUS_EngineBasic] -> Bus Creator/3
  [ASMBUS_VehicleDynamics] -> Bus Creator/2
